simulink model "Controller1"  (R2024a)
settings: Solver=FixedStepAuto  StartTime=0.0  StopTime=10.0  RelTol=1e-3
libraries: robotlib x5
settings Model: Creator=ellanelson  LastModifiedBy=katiegildersleeve
settings OptimizationCC: EnhancedBackFolding=on  PassReuseOutputArgsAs=Individual arguments  ZeroExternalMemoryAtStartup=off  ZeroInternalMemoryAtStartup=off  MaxStackSize=64  OptimizeBlockOrder=speed  DifferentSizesBufferReuse=on  OptimizationCustomize=off  EfficientTunableParamExpr=on
settings DebuggingCC: ParameterTunabilityLossMsg=error
settings HardwareCC: ProdBitPerPointer=32  ProdBitPerSizeT=32  ProdBitPerPtrDiffT=32  ProdLargestAtomicFloat=None  ProdIntDivRoundTo=Undefined  ProdEndianess=Unspecified  ProdWordSize=32  ProdHWDeviceType=Generic->Unspecified (assume 32-bit Generic)  UseEmbeddedCoderFeatures=off  UseSimulinkCoderFeatures=off
settings SFSimCC: MATLABDynamicMemAlloc=off
settings RTWCC: Description=Embedded Coder  SystemTargetFile=ert.tlc  HardwareBoard=Robot Operating System (ROS)  TLCOptions="-aInlineSetEventsForThisBaseRateFcn=TLC_FALSE -aSuppressMultiTaskScheduler=TLC_FALSE  -aRateBasedStepFcn=0"  TemplateMakefile=ert_default_tmf  Toolchain=Catkin  TargetLang=C++
settings CodeAppCC: ForceParamTrailComments=on  IgnoreCustomStorageClasses=off  OperatorAnnotations=on  SimulinkDataObjDesc=on  SFDataObjDesc=on  InsertBlockDesc=on
settings ERTTargetCC: SupportNonInlinedSFcns=on

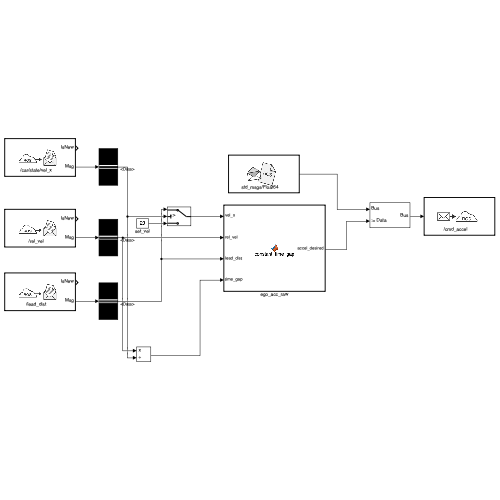
[thumbnail: Simulink's stored preview of the top-level diagram]
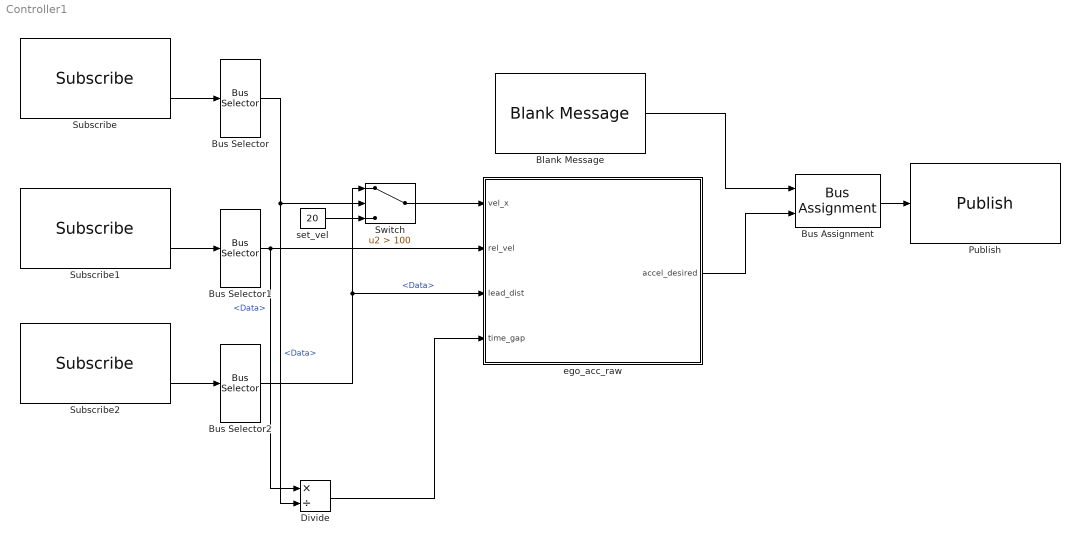
== system Controller1 ==
  Blank Message : robotlib/Blank Message  messageClass=Message  entityType=std_msgs/Float64  messageType=std_msgs/Float64  SampleTime=inf  legacyBusStruct=off
  Bus Assignment : BusAssignment  AssignedSignals=Data
  Bus Selector : BusSelector  OutputSignals=Data
  Bus Selector1 : BusSelector  OutputSignals=Data
  Bus Selector2 : BusSelector  OutputSignals=Data
  Divide : Product  Inputs=*/
  Publish : robotlib/Publish  topicSource=Specify your own  topic=/cmd_accel  messageType=std_msgs/Float64  legacyBusStruct=off  messageQueueLength=1
  Subscribe : robotlib/Subscribe  topicSource=Specify your own  topic=/car/state/vel_x  messageType=std_msgs/Float64  SampleTime=-1  legacyBusStruct=off  messageQueueLength=1
  Subscribe1 : robotlib/Subscribe  topicSource=Specify your own  topic=/rel_vel  messageType=std_msgs/Float64  SampleTime=-1  legacyBusStruct=off  messageQueueLength=1
  Subscribe2 : robotlib/Subscribe  topicSource=Specify your own  topic=/lead_dist  messageType=std_msgs/Float64  SampleTime=-1  legacyBusStruct=off  messageQueueLength=1
  Switch : Switch  Criteria=u2 > Threshold  Threshold=100  SaturateOnIntegerOverflow=off  InputSameDT=off
  ego_acc_raw : MATLAB Function  TreatAsAtomicUnit=on
  set_vel : Constant  Value=20
  wires:
  Bus Assignment/1 -> Publish/1
  Blank Message/1 -> Bus Assignment/1
  ego_acc_raw/1(accel_desired) -> Bus Assignment/2
  Subscribe/2 -> Bus Selector/1
  Bus Selector/1 -> Switch/2, Divide/2  "<Data>"
  Subscribe1/2 -> Bus Selector1/1
  Bus Selector1/1 -> ego_acc_raw/2(rel_vel), Divide/1  "<Data>"
  Divide/1 -> ego_acc_raw/4(time_gap)
  Bus Selector2/1 -> ego_acc_raw/3(lead_dist), Switch/1  "<Data>"
  Subscribe2/2 -> Bus Selector2/1
  set_vel/1 -> Switch/3
  Switch/1 -> ego_acc_raw/1(vel_x)

== matlab function Controller1/ego_acc_raw ==
  data: vel_x input; rel_vel input; lead_dist input; accel_desired output; time_gap input
function accel_desired = constant_time_gap(vel_x, rel_vel, lead_dist, time_gap)

% Define the desired time gap and the proportional control gain
tau = time_gap;        
alpha = 1.5;    

% Calculate the desired space gap based on the ego vehicle's speed
s_desired = tau * vel_x;

% Calculate the desired acceleration based on the space gap and speed gap
accel_desired = alpha * ( (lead_dist - s_desired) + rel_vel );
